simulink model "Non_lin_DroneDynam_WithActuator"  (R2024a)
settings: Solver=VariableStepAuto  StartTime=0.0  StopTime=30  RelTol=1e-3
undefined symbols (not defined in the file): aEval, bEval, fxc, fyc, Kp, Kpe, Kphi, Kpn, Kpz, Kq, Kr, Ktheta, Ku, Kv, Kw, Kyaw, mixMat, Pdc, Pec, Pnc, Yawc
settings Model: Creator=achic  LastModifiedBy=achic

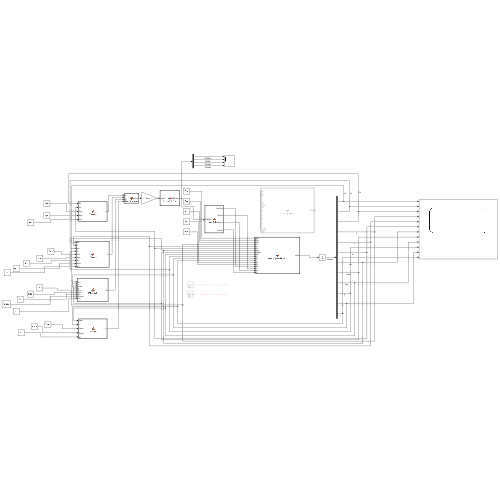
[thumbnail: Simulink's stored preview of the top-level diagram]
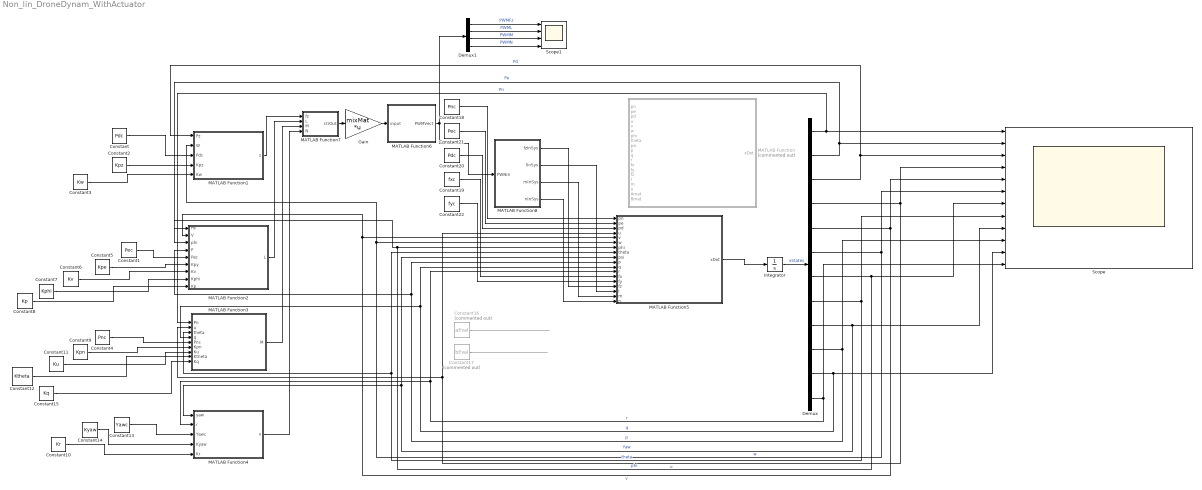
== system Non_lin_DroneDynam_WithActuator ==
  Constant : Constant  Value=Pdc
  Constant1 : Constant  Value=Pec
  Constant10 : Constant  Value=Kr
  Constant11 : Constant  Value=Ku
  Constant12 : Constant  Value=Ktheta
  Constant13 : Constant  Value=Yawc
  Constant14 : Constant  Value=Kyaw
  Constant15 : Constant  Value=Kq
  Constant16 : Constant  Commented=on  Value=aEval
  Constant17 : Constant  Commented=on  Value=bEval
  Constant18 : Constant  Value=Pnc
  Constant19 : Constant  Value=fxc
  Constant2 : Constant  Value=Kpz
  Constant20 : Constant  Value=Pdc
  Constant21 : Constant  Value=Pec
  Constant22 : Constant  Value=fyc
  Constant3 : Constant  Value=Kw
  Constant4 : Constant  Value=Pnc
  Constant5 : Constant  Value=Kpe
  Constant6 : Constant  Value=Kv
  Constant7 : Constant  Value=Kphi
  Constant8 : Constant  Value=Kp
  Constant9 : Constant  Value=Kpn
  Demux : Demux  Outputs=12
  Demux1 : Demux
  Gain : Gain  Gain=mixMat  Multiplication=Matrix(K*u)
  Integrator : Integrator
  MATLAB Function : MATLAB Function  Commented=on  TreatAsAtomicUnit=on
  MATLAB Function1 : MATLAB Function  TreatAsAtomicUnit=on
  MATLAB Function2 : MATLAB Function  TreatAsAtomicUnit=on
  MATLAB Function3 : MATLAB Function  TreatAsAtomicUnit=on
  MATLAB Function4 : MATLAB Function  TreatAsAtomicUnit=on
  MATLAB Function5 : MATLAB Function  TreatAsAtomicUnit=on
  MATLAB Function6 : MATLAB Function  TreatAsAtomicUnit=on
  MATLAB Function7 : MATLAB Function  TreatAsAtomicUnit=on
  MATLAB Function8 : MATLAB Function  TreatAsAtomicUnit=on
  Scope : Scope  NumInputPorts=12
  Scope1 : Scope  NumInputPorts=4
  wires:
  MATLAB Function8/2(lInSys) -> MATLAB Function5/16(l)
  Constant5/1 -> MATLAB Function2/6(Kpy)
  Constant7/1 -> MATLAB Function2/8(Kphi)
  MATLAB Function3/1(M) -> MATLAB Function7/3(M)
  MATLAB Function4/1(n) -> MATLAB Function7/4(N)
  Constant8/1 -> MATLAB Function2/9(Kp)
  Demux/2 -> MATLAB Function2/1(Pe), Scope/2  "Pe"
  MATLAB Function8/3(mInSys) -> MATLAB Function5/17(m)
  Demux/9 -> Scope/9, MATLAB Function5/9(psi), MATLAB Function4/1(yaw)  "Yaw"
  Constant14/1 -> MATLAB Function4/4(Kyaw)
  Demux/1 -> MATLAB Function3/1(Pn), Scope/1  "Pn"
  MATLAB Function8/1(fzInSys) -> MATLAB Function5/15(fz)
  Constant16/1 -> ?
  Constant6/1 -> MATLAB Function2/7(Kv)
  Demux/11 -> Scope/11, MATLAB Function5/11(q), MATLAB Function3/4(q)  "q"
  Demux/3 -> MATLAB Function1/1(Pz), Scope/3  "Pd"
  MATLAB Function5/1(xDot) -> Integrator/1
  Constant17/1 -> ?
  Constant1/1 -> MATLAB Function2/5(Pec)
  Constant20/1 -> MATLAB Function5/3(pd)
  Constant18/1 -> MATLAB Function5/1(pn)
  Gain/1 -> MATLAB Function6/1(input)
  Constant15/1 -> MATLAB Function3/9(Kq)
  MATLAB Function1/1(z) -> MATLAB Function7/1(fz)
  Demux1/3 -> Scope1/3  "PWMM"
  Constant22/1 -> MATLAB Function5/14(fy)
  Demux1/2 -> Scope1/2  "PWML"
  Demux/12 -> MATLAB Function5/12(r), MATLAB Function4/2(r), Scope/12  "r"
  Demux/4 -> MATLAB Function5/4(u), MATLAB Function3/2(u), Scope/4  "u"
  Demux/8 -> Scope/8, MATLAB Function5/8(theta), MATLAB Function3/3(theta)  "theta"
  Constant19/1 -> MATLAB Function5/13(fx)
  Demux/10 -> Scope/10, MATLAB Function5/10(p), MATLAB Function2/4(P)  "p"
  Constant/1 -> MATLAB Function1/3(Pdc)
  MATLAB Function8/4(nInSys) -> MATLAB Function5/18(n)
  Constant4/1 -> MATLAB Function3/5(Pnc)
  Demux/5 -> Scope/5, MATLAB Function5/5(v), MATLAB Function2/2(V)  "v"
  Demux/7 -> Scope/7, MATLAB Function5/7(phi), MATLAB Function2/3(phi)  "phi"
  Demux1/1 -> Scope1/1  "PWMFz"
  MATLAB Function6/1(PWMVect) -> Demux1/1, MATLAB Function8/1(PWNIn)
  Constant12/1 -> MATLAB Function3/8(Ktheta)
  Constant10/1 -> MATLAB Function4/5(Kr)
  Demux1/4 -> Scope1/4  "PWMN"
  MATLAB Function7/1(ctrOut) -> Gain/1
  Constant2/1 -> MATLAB Function1/4(Kpz)
  Integrator/1 -> Demux/1  "xStates"
  MATLAB Function2/1(L) -> MATLAB Function7/2(L)
  Constant9/1 -> MATLAB Function3/6(Kpn)
  Constant3/1 -> MATLAB Function1/5(Kw)
  Demux/6 -> Scope/6, MATLAB Function5/6(w), MATLAB Function1/2(W)  "w"
  Constant21/1 -> MATLAB Function5/2(pe)
  Constant13/1 -> MATLAB Function4/3(Yawc)
  Constant11/1 -> MATLAB Function3/7(Ku)

== matlab function Non_lin_DroneDynam_WithActuator/MATLAB Function5 ==
  data: pn input; pe input; pd input; u input; xDot output; v input; w input; phi input; theta input; psi input; p input; q input; r input; fx input; fy input; fz input; l input; m input; n input
function xDot = DroneDynamNonLin(pn, pe, pd, u, v, w, phi, theta, psi, p, q, r, fx, fy, fz, l, m, n)
    mass = 0.033; % Units = kg. Mass of drone.
    g = 9.8; % m/s^2.

    cTheta = cosd(theta);
    cPhi = cosd(phi);
    cPsi = cosd(psi);
    
    sTheta = sind(theta);
    sPhi = sind(phi);
    sPsi = sind(psi);
    
    tTheta = tand(theta);
    
    
    
    %inerMatrix = Jy * eye(3); % Inertial Tensor matrix.
    inerMatrix = [16.57,  0.83,  0.72;
                   0.83, 16.66,  1.80;
                   0.72,  1.80, 29.26]; % Inertial Tensor matrix. In the body frame.
    
    Jx = inerMatrix(1, 1);
    Jxy = inerMatrix(2, 1);
    Jxz = inerMatrix(3, 1);
    %Jxy = inerMatrix(1, 2);
    Jy = inerMatrix(2, 2);
    Jyz = inerMatrix(3, 2);
    %Jxz = inerMatrix(1, 3);
    %Jyz = inerMatrix(2, 3);
    Jz = inerMatrix(3, 3);
    
    tau = Jx * Jz - Jxz^2;
    Tau1 = (Jxz * (Jx - Jy + Jz) ) / tau;
    Tau2 = (Jz * (Jz - Jy) + Jxz^2 ) / tau;
    Tau3 = Jz / tau;
    Tau4 = Jxz / tau;
    Tau5 = (Jz - Jx) / Jy;
    Tau6 = Jxz / Jy;
    Tau7 = ( (Jx - Jy) * Jx + Jxz^2) / tau;
    Tau8 = Jx / tau;
    % Creating the system of equations and putting it into a column vector.
    xDot = [(cTheta * cPsi) * u + (sPhi * sTheta * cPsi - cPhi * sPsi) * v + (cPhi * sTheta * cPsi + sPhi * sPsi)* w;
         (cTheta * sPsi) * u + (sPhi * sTheta * sPsi + cPhi * cPsi) * v + (cPhi * sTheta* sPsi - sPhi * cPsi) * w;
         (-sTheta) * u + (sPhi * cTheta) * v + (cPhi * cTheta) * w;
         r * v - q * w + fx / mass;
         p * w - r * u + fy / mass;
         q * u - p * v + fz / mass;
         p + (sPhi * tTheta) * q + (cPhi * tTheta) * r;
         0 + cPhi * q - sPhi * r;
         0 + (sPhi / cTheta) * q + (cPhi / cTheta) * r;
         (Tau1 * p * q - Tau2 * q * r) + Tau3 * l + Tau4 * n;
         Tau5 * p * r - Tau6 * (p^2 - r^2) + (1 / Jy) * m;
         Tau7 * p * q - Tau1 * q * r + Tau4 * l + Tau8 * n];
end

== matlab function Non_lin_DroneDynam_WithActuator/MATLAB Function6 ==
  data: input input; PWMVect output
function PWMVect = ThrustToPWM(input)

    fz = input(1);
    L = input(2);
    M = input(3);
    N = input(3);
    momentArmLeng = 0.046; % Units meters.
    
    PWMFromThrustFunc = @(thrust) (77371252455336267181195264 * sqrt(3296015354597325 * thrust / 38685626227668133590597632 + 182045336161068188949327330602267/178405961588244985132285746181186892047843328) / 3296015354597325 -  79924503786362355712/3296015354597325);
    
    PWMFromTorFunc = @(tor)  (19807040628566084398385987584 * sqrt(5032769273675311 * tor / 9903520314283042199192993792 + 663141903269232066005393670573721 / 23384026197294446691258957323460528314494920687616) /  5032769273675311 - 122038747880436514816 / 5032769273675311);

    LTorqForce = L / momentArmLeng; % Thrust force that makes torque L.
    MTorqForce = M / momentArmLeng;
    
    if fz < 0
        PWMFz = 0;
    else
        PWMFz = double(PWMFromThrustFunc(fz));
    end

    if L < 0
        PWML = 0;
    else 
        PWML = double(PWMFromThrustFunc(LTorqForce));
    end
    
    if M < 0
        PWMM = 0;
    else
        PWMM = double(PWMFromThrustFunc(MTorqForce));
    end

    if N < 0
        PWMN = 0;
    else
        PWMN = double(PWMFromTorFunc(N));
    end
    
    PWMVect = [PWMFz, PWML, PWMM, PWMN]';

end

== matlab function Non_lin_DroneDynam_WithActuator/MATLAB Function7 ==
  data: fz input; ctrOut output; L input; M input; N input
function ctrOut = TurnToVector(fz, L, M, N)
    
    
    ctrOut = [fz, L, M, N]';
end

== matlab function Non_lin_DroneDynam_WithActuator/MATLAB Function8 ==
  data: PWNIn input; fzInSys output; lInSys output; mInSys output; nInSys output
function [fzInSys, lInSys, mInSys, nInSys] = ActOnSys(PWNIn)
    A = 2.13* 10 ^ -11; % From Assignment Doc.
    B = 1.033 * 10 ^ -6;
    C = 5.48 * 10 ^ -4;
    D = 0.005964552;
    E = 1.563 * 10 ^ -5;

    momentArmLeng = 0.046; % Units meters.
    equaThrus = @(PWM)  A * PWM^2 + B * PWM + C;
    
    equaTor = @(PWM) D * (A * PWM^2 + B * PWM + C) + E;
    
    
    fzPWM = PWNIn(1);
    LPWM = PWNIn(2);
    MPWM = PWNIn(3);
    NPWM = PWNIn(4);
    
    fzInSys = equaThrus(fzPWM);
    lInSys = momentArmLeng * equaThrus(LPWM);
    mInSys = momentArmLeng * equaThrus(MPWM);
    nInSys = equaTor(NPWM);
end

== matlab function Non_lin_DroneDynam_WithActuator/MATLAB Function1 ==
  data: Pz input; z output; W input; Pdc input; Kpz input; Kw input
function z = ZControl(Pz, W, Pdc, Kpz, Kw)
    % Using NED 
    K = [Pdc * Kpz * Kw, -Kpz * Kw, -Kw];
    stateVec = [1, Pz, W]';
    z = K * stateVec; 
end

== matlab function Non_lin_DroneDynam_WithActuator/MATLAB Function ==
  data: pn input; pe input; pd input; u input; xDot output; v input; w input; phi input; theta input; psi input; p input; q input; r input; fx input; fy input; fz input; l input; m input; n input; Amat input; Bmat input
function xDot = DroneDynamLin(pn, pe, pd, u, v, w, phi, theta, psi, p, q, r, fx, fy, fz, l, m, n, Amat, Bmat)
    xVec = [pn, pe, pd, u, v, w, phi, theta, psi, p, q, r]';
    uVec = [fx, fy, fz, l, m, n]';
    xDot = Amat * xVec + Bmat * uVec;
end

== matlab function Non_lin_DroneDynam_WithActuator/MATLAB Function2 ==
  data: L output; Pe input; V input; phi input; P input; Pec input; Kpy input; Kv input; Kphi input; Kp input
function L = LControl(Pe, V, phi, P, Pec, Kpy, Kv, Kphi, Kp)
    K = [Pec * Kpy * Kv * Kphi * Kp, -Kpy * Kv * Kphi * Kp, -Kv * Kphi * Kp, -Kphi * Kp, -Kp];
    stateVec = [1, Pe, V, phi, P]';
    L = K * stateVec; 
end

== matlab function Non_lin_DroneDynam_WithActuator/MATLAB Function3 ==
  data: Pn input; u input; M output; theta input; q input; Pnc input; Kpn input; Ku input; Ktheta input; Kq input
function M = MControl(Pn, u, theta, q, Pnc, Kpn, Ku, Ktheta, Kq)
    K = [Pnc * Kpn * Ku * Ktheta * Kq, -Kpn *Ku * Ktheta * Kq, -Ku * Ktheta * Kq, -Ktheta * Kq, -Kq];
    stateVec = [1, Pn, u, theta, q]';
    M = K * stateVec; 
end

== matlab function Non_lin_DroneDynam_WithActuator/MATLAB Function4 ==
  data: yaw input; n output; r input; Yawc input; Kyaw input; Kr input
function n = NControl(yaw, r, Yawc, Kyaw, Kr)
    K = [Yawc * Kyaw * Kr, -Kyaw * Kr, -Kr];
    stateVec = [1, yaw, r]';
    n = K * stateVec; 
end
